simulink model "trafficlight"  (R2015a)
settings: Solver=FixedStepDiscrete  SolverMode=SingleTasking  StartTime=0.0  StopTime=10.0  RelTol=1e-3
settings Model: CovSFcnEnable=off  Creator=3w09  LastModifiedBy=Keshav
settings DebuggingCC: SolverPrmCheckMsg=warning

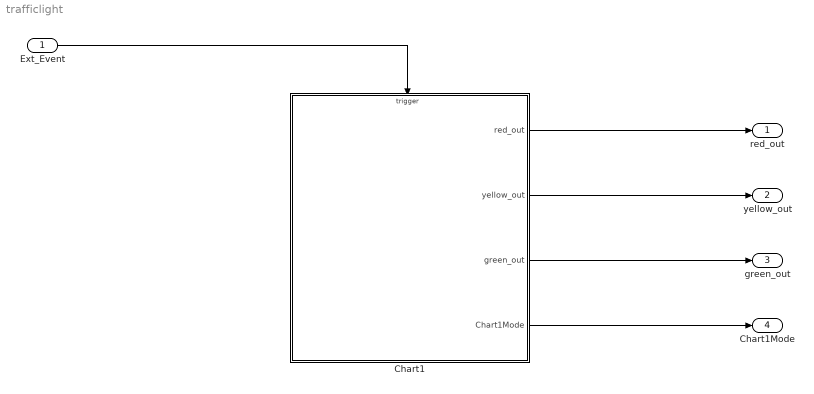
== system trafficlight ==
  Ext_Event : Inport
  Chart1 : Stateflow chart  TreatAsAtomicUnit=on
  red_out : Outport
  yellow_out : Outport  Port=2
  green_out : Outport  Port=3
  Chart1Mode : Outport  Port=4
  wires:
  Ext_Event/1 -> Chart1/Trigger
  Chart1/1(red_out) -> red_out/1
  Chart1/2(yellow_out) -> yellow_out/1
  Chart1/3(green_out) -> green_out/1
  Chart1/4(Chart1Mode) -> Chart1Mode/1

== stateflow chart trafficlight/Chart1 ==
  state R
    entry: red_out = 1;
    during: red_out = 1;
    exit: red_out = 0;
  state Y
    entry: yellow_out = 1;
    exit: yellow_out = 0;
  state G
    entry: green_out = 1;
    exit: green_out = 0;
  (default) -> R
  Y -> R : after(2, sec)
  R -> G : go_cmd
  G -> Y : after(3, sec)
  data: red_out output; yellow_out output; green_out output; Chart1Mode output Enum: Chart1ModeType
  events: master_trigger input EITHER_EDGE_EVENT; go_cmd input RISING_EDGE_EVENT
